simulink model "Combined_Experiment_Mar25_2020a_SpeedControl"  (R2020a)
settings: Solver=FixedStepAuto  StartTime=0.0  StopTime=tsim  FixedStep=baseRate  MaxStep=0.0001  RelTol=1e-6  AbsTol=1e-6  EnableMultiTasking=on
values from neighbouring files (symbols this model uses):
  b0 = importdata("biases_layer_0.csv")    [Run_Initializer.m]
  b1 = importdata("biases_layer_1.csv")    [Run_Initializer.m]
  b_out = importdata("biases_output.csv")    [Run_Initializer.m]
  baseRate = 0.05    [Run_Initializer.m]
  CHASER_ABSOLUTE_POSITION = true    [Run_Initializer.m]
  drop_states_ARM = [ pi/2, pi/2, 0]    [Run_Initializer.m]
  drop_states_BLACK = [ xLength/2, yLength/2, pi]    [Run_Initializer.m]
  drop_states_BLUE = [ xLength/2, yLength/2, pi]    [Run_Initializer.m]
  drop_states_RED = [ xLength/2+0.5, yLength/2, pi]    [Run_Initializer.m]
  F_Black_X_nominal = 0.2196    [Run_Initializer.m]
  F_Black_Y_nominal = 0.2825    [Run_Initializer.m]
  F_Blue_X_nominal = 0.2196    [Run_Initializer.m]
  F_Blue_Y_nominal = 0.2825    [Run_Initializer.m]
  F_red_X_nominal = 0.2196    [Run_Initializer.m]
  F_red_Y_nominal = 0.2825    [Run_Initializer.m]
  F_thrusters_BLACK = [F_Black_X_nominal; F_Black_X_nominal;                             F_Black_Y_nominal; F_Black_Y_nominal; F_Black_X_nominal;                              F_Black_X_nominal; F_Black_Y_nominal; F_Black_Y_nominal]    [Run_Initializer.m]
  F_thrusters_BLUE = [F_Blue_X_nominal; F_Blue_X_nominal;                             F_Blue_Y_nominal; F_Blue_Y_nominal; F_Blue_X_nominal;                              F_Blue_X_nominal; F_Blue_Y_nominal; F_Blue_Y_nominal]    [Run_Initializer.m]
  F_thrusters_RED = [F_red_X_nominal; F_red_X_nominal;                             F_red_Y_nominal; F_red_Y_nominal; F_red_X_nominal;                              F_red_X_nominal; F_red_Y_nominal; F_red_Y_nominal]    [Run_Initializer.m]
  Gamma1_el = 0.12    [Run_Initializer.m]
  Gamma1_sh = 0.005    [Run_Initializer.m]
  Gamma1_wr = 0.025    [Run_Initializer.m]
  Gamma2_el = 5    [Run_Initializer.m]
  Gamma2_sh = 15    [Run_Initializer.m]
  Gamma2_wr = 5    [Run_Initializer.m]
  Gamma3_el = 10    [Run_Initializer.m]
  Gamma3_sh = 40    [Run_Initializer.m]
  Gamma3_wr = 40    [Run_Initializer.m]
  Gamma4_el = 0.039    [Run_Initializer.m]
  Gamma4_sh = 0.015    [Run_Initializer.m]
  Gamma4_wr = 0.029    [Run_Initializer.m]
  Gamma5_el = 800    [Run_Initializer.m]
  Gamma5_sh = 800    [Run_Initializer.m]
  Gamma5_wr = 800    [Run_Initializer.m]
  Gamma6_el = 0.000001    (= 1e-06)    [Run_Initializer.m]
  Gamma6_sh = 0.005    [Run_Initializer.m]
  Gamma6_wr = 0.02    [Run_Initializer.m]
  HOLD_POINT_RADIUS = 0.95    [Run_Initializer.m]
  home_states_BLACK = [ xLength/2; yLength/2; 0]    [Run_Initializer.m]
  home_states_BLUE = [ xLength/2; yLength/2; 0]    [Run_Initializer.m]
  home_states_RED = [ xLength/2+0.9; yLength/2; pi]    [Run_Initializer.m]
  init_states_BLACK = [ xLength/2; yLength/2; pi]    [Run_Initializer.m]
  init_states_BLUE = [ xLength/2; yLength/2; pi]    [Run_Initializer.m]
  init_states_RED = [ xLength/2+0.9; yLength/2; pi]    [Run_Initializer.m]
  Kd_tb = 1.0    (= 1)    [Run_Initializer.m]
  Kd_tblue = 1    [Run_Initializer.m]
  Kd_tr = 1.0    (= 1)    [Run_Initializer.m]
  Kd_xb = 8    [Run_Initializer.m]
  Kd_xblue = 8    [Run_Initializer.m]
  Kd_xr = 8    [Run_Initializer.m]
  Kd_yb = 8    [Run_Initializer.m]
  Kd_yblue = 8    [Run_Initializer.m]
  Kd_yr = 8    [Run_Initializer.m]
  Kp_tb = 0.1    [Run_Initializer.m]
  Kp_tblue = 0.1    [Run_Initializer.m]
  Kp_tr = 0.1    [Run_Initializer.m]
  Kp_xb = 2    [Run_Initializer.m]
  Kp_xblue = 2    [Run_Initializer.m]
  Kp_xr = 2    [Run_Initializer.m]
  Kp_yb = 2    [Run_Initializer.m]
  Kp_yblue = 2    [Run_Initializer.m]
  Kp_yr = 2    [Run_Initializer.m]
  MAX_BODY_ANGULAR_VELOCITY = 15*180/pi    (= 859.436692696)    [Run_Initializer.m]
  MAX_VELOCITY = 0.1    [Run_Initializer.m]
  noise_variance_BLACK = 0    [Run_Initializer.m]
  noise_variance_BLUE = 0    [Run_Initializer.m]
  noise_variance_RED = 0    [Run_Initializer.m]
  Phase0_End = Phase0_Duration    (= 10)    [Run_Initializer.m]
  Phase1_End = Phase0_Duration + Phase1_Duration    (= 15)    [Run_Initializer.m]
  Phase2_End = Phase0_Duration + Phase1_Duration +                                   Phase2_Duration    (= 45)    [Run_Initializer.m]
  Phase3_End = Phase0_Duration + Phase1_Duration +                                   Phase2_Duration + Phase3_Duration    (= 560)    [Run_Initializer.m]
  Phase3_SubPhase1_End = Phase2_End + Phase3_SubPhase1_Duration    (= 105)    [Run_Initializer.m]
  Phase3_SubPhase2_End = Phase2_End + Phase3_SubPhase1_Duration +                                   Phase3_SubPhase2_Duration    (= 210)    [Run_Initializer.m]
  Phase3_SubPhase3_End = Phase2_End + Phase3_SubPhase1_Duration +                                   Phase3_SubPhase2_Duration +                                  Phase3_SubPhase3_Duration    (= 240)    [Run_Initializer.m]
  Phase3_SubPhase4_End = Phase2_End + Phase3_SubPhase1_Duration +                                   Phase3_SubPhase2_Duration +                                  Phase3_SubPhase3_Duration +                                  Phase3_SubPhase4_Duration    [Run_Initializer.m]
  Phase4_End = Phase0_Duration + Phase1_Duration +                                   Phase2_Duration + Phase3_Duration +                                   Phase4_Duration    (= 680)    [Run_Initializer.m]
  Phase5_End = Phase0_Duration + Phase1_Duration +                                   Phase2_Duration + Phase3_Duration +                                   Phase4_Duration + Phase5_Duration    (= 700)    [Run_Initializer.m]
  relevant_half_range = (upper_state_bound - lower_state_bound)/2    [Run_Initializer.m]
  relevant_state_mean = (lower_state_bound + upper_state_bound)/2    [Run_Initializer.m]
  thruster_dist2CG_BLACK = [72.80;-65.20;61.75;-79.75;65.20;-65.20;74.25;-54.75]    [Run_Initializer.m]
  thruster_dist2CG_BLUE = [83.10;-54.90;71.50;-70.00;54.90;-75.50;64.50;-64.50]    [Run_Initializer.m]
  thruster_dist2CG_RED = [69.38;-56.62;50.01;-81.49;61.12;-68.38;78.99;-52.01]    [Run_Initializer.m]
  w0 = importdata("weights_layer_0.csv")    [Run_Initializer.m]
  w1 = importdata("weights_layer_1.csv")    [Run_Initializer.m]
  w_out = importdata("weights_output.csv")    [Run_Initializer.m]
  xLength = 3.51155    [Run_Initializer.m]
  yLength = 2.41935    [Run_Initializer.m]
undefined symbols (not defined in the file or in its folder): DiscIntNeverNeededParam, model_param, platformSelection, serverRate, simMode
libraries: dspstat3 x18, raspberrypiBasiclib x9, dspsigops x9, simulink x8, embdlinuxlib x7, MainLibrary x4, mspfiltlib x3, dsparch4 x3, etargetslib x1, sensehatlib x1
(part 8 of 13)

== system Combined_Experiment_Mar25_2020a_SpeedControl/Phase #3: Experiment/Change RED Behavior/Sub-Phase #3 /RED+ARM ==
  note: ARM Control Law - RED
  note: This section is reserved for any control law for the robotic manipulator.
  Action Port : ActionPort  ActionPortLabel=if(u1 == 4 | u1 == 5 | u1 == 10 | u1 == 11)
  1-D Lookup Table : Lookup_n-D  NumberOfTableDimensions=1  BreakpointsForDimension1=|  Table=|  InternalRulePriority=Speed  RndMeth=Simplest  InputSameDT=on
      BreakpointsForDimension1=|
      | [0
      | 0.300000000000000
      | 0.600000000000000
      | 0.900000000000000
      | 1.20000000000000
      | 1.50000000000000
      | 1.80000000000000
      | 2.10000000000000
      | 2.40000000000000
      | 2.70000000000000
      | 3
      | 3.30000000000000
      | 3.60000000000000
      | 3.90000000000000
      | 4.20000000000000
      | 4.50000000000000
      | 4.80000000000000
      | 5.10000000000000
      | 5.40000000000000
      | 5.70000000000000
      | 6
      | 6.30000000000000
      | 6.60000000000000
      | 6.90000000000000
      | 7.20000000000000
      | 7.50000000000000
      | 7.80000000000000
      | 8.10000000000000
      | 8.40000000000000
      | 8.70000000000000
      | 9
      | 9.30000000000000
      | 9.60000000000000
      | 9.90000000000000
      | 10.2000000000000
      | 10.5000000000000
      | 10.8000000000000
      | 11.1000000000000
      | 11.4000000000000
      | 11.7000000000000
      | 12
      | 12.3000000000000
      | 12.6000000000000
      | 12.9000000000000
      | 13.2000000000000
      | 13.5000000000000
      | 13.8000000000000
      | 14.1000000000000
      | 14.4000000000000
      | 14.7000000000000
      | 15
      | 15.3000000000000
      | 15.6000000000000
      | 15.9000000000000
      | 16.2000000000000
      | 16.5000000000000
      | 16.8000000000000
      | 17.1000000000000
      | 17.4000000000000
      | 17.7000000000000
      | 18
      | 18.3000000000000
      | 18.6000000000000
      | 18.9000000000000
      | 19.2000000000000
      | 19.5000000000000
      | 19.8000000000000
      | 20.1000000000000
      | 20.4000000000000
      | 20.7000000000000
      | 21
      | 21.3000000000000
      | 21.6000000000000
      | 21.9000000000000
      | 22.2000000000000
      | 22.5000000000000
      | 22.8000000000000
      | 23.1000000000000
      | 23.4000000000000
      | 23.7000000000000
      | 24
      | 24.3000000000000
      | 24.6000000000000
      | 24.9000000000000
      | 25.2000000000000
      | 25.5000000000000
      | 25.8000000000000
      | 26.1000000000000
      | 26.4000000000000
      | 26.7000000000000
      | 27
      | 27.3000000000000
      | 27.6000000000000
      | 27.9000000000000
      | 28.2000000000000
      | 28.5000000000000
      | 28.8000000000000
      | 29.1000000000000
      | 29.4000000000000
      | 29.7000000000000
      | 30]
      Table=|
      | [1.57000000000000
      | 1.54816700100684
      | 1.49097838714515
      | 1.40738374526561
      | 1.30517963261499
      | 1.19037595061406
      | 1.06817443571262
      | 0.943755752477061
      | 0.821348547944454
      | 0.703746844506339
      | 0.593625926874354
      | 0.493661079760138
      | 0.406301951764504
      | 0.332150464577563
      | 0.270904238844892
      | 0.222254718367453
      | 0.185893346946205
      | 0.161510391400890
      | 0.148507079640713
      | 0.145619174532266
      | 0.151489118608687
      | 0.164759354403110
      | 0.184072324448674
      | 0.208070471278512
      | 0.235433340233479
      | 0.265163793185692
      | 0.296431328827974
      | 0.328406827894775
      | 0.360261171120541
      | 0.391165239239719
      | 0.420289912986756
      | 0.446835197706220
      | 0.470407808441224
      | 0.490913309071205
      | 0.508264171683338
      | 0.522372868364801
      | 0.533151871202771
      | 0.540513652284423
      | 0.544370683696935
      | 0.544708678506983
      | 0.541826697403650
      | 0.536107583537685
      | 0.527934180942696
      | 0.517689333652287
      | 0.505755885700064
      | 0.492516681119634
      | 0.478354564411779
      | 0.463677280032886
      | 0.448984347405091
      | 0.434796424940426
      | 0.421634171050923
      | 0.410018244148617
      | 0.400469302645538
      | 0.393508004953720
      | 0.389655009485195
      | 0.389318793355856
      | 0.392420798366228
      | 0.398750326166947
      | 0.408096675929411
      | 0.420249146825022
      | 0.434997038025178
      | 0.452129648701280
      | 0.471436276672662
      | 0.492577909508950
      | 0.514735652583953
      | 0.536978444975800
      | 0.558375225762617
      | 0.577994934022531
      | 0.594906508833669
      | 0.608178889274159
      | 0.616885200503004
      | 0.620279657398225
      | 0.617862923664403
      | 0.609153311284521
      | 0.593669132241562
      | 0.570928698518508
      | 0.540450322098342
      | 0.501754708369804
      | 0.454651142688837
      | 0.399508826722755
      | 0.336761216407457
      | 0.266841767678842
      | 0.190183936472810
      | 0.107221178725261
      | 0.0184637402812976
      | -0.0750305460272099
      | -0.171966007758580
      | -0.271046003976081
      | -0.370973893742981
      | -0.470452548764951
      | -0.568113490727538
      | -0.662442454298735
      | -0.751907371290790
      | -0.834976173515947
      | -0.910130221885170
      | -0.976013131751286
      | -1.03137619058426
      | -1.07497442671845
      | -1.10593044052833
      | -1.12417944460303
      | -1.20000000000000]
  1-D Lookup Table1 : Lookup_n-D  NumberOfTableDimensions=1  BreakpointsForDimension1=|  Table=|  InternalRulePriority=Speed  RndMeth=Simplest  InputSameDT=on
      BreakpointsForDimension1=|
      | [0
      | 0.300000000000000
      | 0.600000000000000
      | 0.900000000000000
      | 1.20000000000000
      | 1.50000000000000
      | 1.80000000000000
      | 2.10000000000000
      | 2.40000000000000
      | 2.70000000000000
      | 3
      | 3.30000000000000
      | 3.60000000000000
      | 3.90000000000000
      | 4.20000000000000
      | 4.50000000000000
      | 4.80000000000000
      | 5.10000000000000
      | 5.40000000000000
      | 5.70000000000000
      | 6
      | 6.30000000000000
      | 6.60000000000000
      | 6.90000000000000
      | 7.20000000000000
      | 7.50000000000000
      | 7.80000000000000
      | 8.10000000000000
      | 8.40000000000000
      | 8.70000000000000
      | 9
      | 9.30000000000000
      | 9.60000000000000
      | 9.90000000000000
      | 10.2000000000000
      | 10.5000000000000
      | 10.8000000000000
      | 11.1000000000000
      | 11.4000000000000
      | 11.7000000000000
      | 12
      | 12.3000000000000
      | 12.6000000000000
      | 12.9000000000000
      | 13.2000000000000
      | 13.5000000000000
      | 13.8000000000000
      | 14.1000000000000
      | 14.4000000000000
      | 14.7000000000000
      | 15
      | 15.3000000000000
      | 15.6000000000000
      | 15.9000000000000
      | 16.2000000000000
      | 16.5000000000000
      | 16.8000000000000
      | 17.1000000000000
      | 17.4000000000000
      | 17.7000000000000
      | 18
      | 18.3000000000000
      | 18.6000000000000
      | 18.9000000000000
      | 19.2000000000000
      | 19.5000000000000
      | 19.8000000000000
      | 20.1000000000000
      | 20.4000000000000
      | 20.7000000000000
      | 21
      | 21.3000000000000
      | 21.6000000000000
      | 21.9000000000000
      | 22.2000000000000
      | 22.5000000000000
      | 22.8000000000000
      | 23.1000000000000
      | 23.4000000000000
      | 23.7000000000000
      | 24
      | 24.3000000000000
      | 24.6000000000000
      | 24.9000000000000
      | 25.2000000000000
      | 25.5000000000000
      | 25.8000000000000
      | 26.1000000000000
      | 26.4000000000000
      | 26.7000000000000
      | 27
      | 27.3000000000000
      | 27.6000000000000
      | 27.9000000000000
      | 28.2000000000000
      | 28.5000000000000
      | 28.8000000000000
      | 29.1000000000000
      | 29.4000000000000
      | 29.7000000000000
      | 30]
      Table=|
      | [1.57000000000000
      | 1.57050205302399
      | 1.57012603662556
      | 1.56661162770156
      | 1.55794488562962
      | 1.54285929753597
      | 1.52042643744410
      | 1.48973080887809
      | 1.45048425411524
      | 1.40334397159352
      | 1.34904540279350
      | 1.28832398919572
      | 1.22195859634965
      | 1.15108368811919
      | 1.07700776270488
      | 1.00104050705195
      | 0.924491608105622
      | 0.848670299127955
      | 0.774774399465782
      | 0.703745216061739
      | 0.636488084287358
      | 0.573908339514172
      | 0.516911317113714
      | 0.466402352457517
      | 0.423202448662068
      | 0.387397731516399
      | 0.358695572215780
      | 0.336800200665272
      | 0.321415846769937
      | 0.312246740434836
      | 0.308997111565029
      | 0.311335869993361
      | 0.318438699519253
      | 0.329118863211428
      | 0.342181246399115
      | 0.356430734411547
      | 0.370672212577955
      | 0.383710566227569
      | 0.394350680689622
      | 0.401518359647600
      | 0.404656733001405
      | 0.403347252632020
      | 0.397171371877986
      | 0.385710544077849
      | 0.368546222570152
      | 0.345259860693440
      | 0.315432914518483
      | 0.278792464474893
      | 0.235602325706072
      | 0.186249942164213
      | 0.131122757801505
      | 0.0706082165701402
      | 0.00509376242231024
      | -0.0650331606897945
      | -0.139385108813982
      | -0.217505825480346
      | -0.298640304539486
      | -0.381952484472539
      | -0.466606302239867
      | -0.551765694801835
      | -0.636594599118806
      | -0.720256952151143
      | -0.801916690711806
      | -0.880723763116082
      | -0.955775800494991
      | -1.02615820551012
      | -1.09095638082305
      | -1.14925572909537
      | -1.20014165298867
      | -1.24269955516454
      | -1.27602769714638
      | -1.29978061439030
      | -1.31436988730625
      | -1.32026130853269
      | -1.31792067070809
      | -1.30781376647092
      | -1.29040638845964
      | -1.26616853457129
      | -1.23607724309064
      | -1.20209333571039
      | -1.16629053007224
      | -1.13074254381788
      | -1.09752309458901
      | -1.06870590002731
      | -1.04630359496360
      | -1.03189323418052
      | -1.02686268208325
      | -1.03259903268412
      | -1.05048937999544
      | -1.08191093831646
      | -1.12679451437392
      | -1.18211552054693
      | -1.24448846973170
      | -1.31052787482445
      | -1.37689087303085
      | -1.44074960138572
      | -1.49961795103105
      | -1.55095978791926
      | -1.58081445088490
      | -1.54996443310863
      | -1.48000000000000]
  1-D Lookup Table2 : Lookup_n-D  NumberOfTableDimensions=1  BreakpointsForDimension1=|  Table=|  InternalRulePriority=Speed  RndMeth=Simplest  InputSameDT=on
      BreakpointsForDimension1=|
      | [0
      | 0.300000000000000
      | 0.600000000000000
      | 0.900000000000000
      | 1.20000000000000
      | 1.50000000000000
      | 1.80000000000000
      | 2.10000000000000
      | 2.40000000000000
      | 2.70000000000000
      | 3
      | 3.30000000000000
      | 3.60000000000000
      | 3.90000000000000
      | 4.20000000000000
      | 4.50000000000000
      | 4.80000000000000
      | 5.10000000000000
      | 5.40000000000000
      | 5.70000000000000
      | 6
      | 6.30000000000000
      | 6.60000000000000
      | 6.90000000000000
      | 7.20000000000000
      | 7.50000000000000
      | 7.80000000000000
      | 8.10000000000000
      | 8.40000000000000
      | 8.70000000000000
      | 9
      | 9.30000000000000
      | 9.60000000000000
      | 9.90000000000000
      | 10.2000000000000
      | 10.5000000000000
      | 10.8000000000000
      | 11.1000000000000
      | 11.4000000000000
      | 11.7000000000000
      | 12
      | 12.3000000000000
      | 12.6000000000000
      | 12.9000000000000
      | 13.2000000000000
      | 13.5000000000000
      | 13.8000000000000
      | 14.1000000000000
      | 14.4000000000000
      | 14.7000000000000
      | 15
      | 15.3000000000000
      | 15.6000000000000
      | 15.9000000000000
      | 16.2000000000000
      | 16.5000000000000
      | 16.8000000000000
      | 17.1000000000000
      | 17.4000000000000
      | 17.7000000000000
      | 18
      | 18.3000000000000
      | 18.6000000000000
      | 18.9000000000000
      | 19.2000000000000
      | 19.5000000000000
      | 19.8000000000000
      | 20.1000000000000
      | 20.4000000000000
      | 20.7000000000000
      | 21
      | 21.3000000000000
      | 21.6000000000000
      | 21.9000000000000
      | 22.2000000000000
      | 22.5000000000000
      | 22.8000000000000
      | 23.1000000000000
      | 23.4000000000000
      | 23.7000000000000
      | 24
      | 24.3000000000000
      | 24.6000000000000
      | 24.9000000000000
      | 25.2000000000000
      | 25.5000000000000
      | 25.8000000000000
      | 26.1000000000000
      | 26.4000000000000
      | 26.7000000000000
      | 27
      | 27.3000000000000
      | 27.6000000000000
      | 27.9000000000000
      | 28.2000000000000
      | 28.5000000000000
      | 28.8000000000000
      | 29.1000000000000
      | 29.4000000000000
      | 29.7000000000000
      | 30]
      Table=|
      | [4.24105195407198e-14
      | 0.00792484586540242
      | 0.0289766808051712
      | 0.0591226460349239
      | 0.0945266677508536
      | 0.132723049258546
      | 0.171865961865416
      | 0.210118613330810
      | 0.245977670299252
      | 0.278442298917847
      | 0.306553255045181
      | 0.329351294539841
      | 0.345978769405532
      | 0.356409999236062
      | 0.361026479142565
      | 0.360212485455902
      | 0.354352294506931
      | 0.343830913350855
      | 0.329212797758318
      | 0.311475554957133
      | 0.291654729751521
      | 0.270785866945703
      | 0.249904511343898
      | 0.230046207750326
      | 0.212190891231227
      | 0.196833909602021
      | 0.184220855187696
      | 0.174595248907400
      | 0.168200611680283
      | 0.165280464425496
      | 0.166078328062186
      | 0.170819192753770
      | 0.179469276510222
      | 0.191804652485855
      | 0.207596998435017
      | 0.226617992112058
      | 0.248639311271326
      | 0.273432633667171
      | 0.300769637053943
      | 0.330372138422153
      | 0.361748634952746
      | 0.394350586665731
      | 0.427629452980086
      | 0.461036693314793
      | 0.494023767088832
      | 0.526042133721183
      | 0.556543253290674
      | 0.585013755003088
      | 0.611069892609436
      | 0.634357776934821
      | 0.654523518804344
      | 0.671213229043108
      | 0.684073018476216
      | 0.692748997928769
      | 0.696887278225870
      | 0.696239394653257
      | 0.691014582997561
      | 0.681546260210274
      | 0.668167845572800
      | 0.651212758366539
      | 0.631014417872893
      | 0.607906243373263
      | 0.582221655279522
      | 0.554401355144190
      | 0.525287277542556
      | 0.495815140112214
      | 0.466920660490759
      | 0.439539556315785
      | 0.414607545224887
      | 0.393060344855659
      | 0.375828988968287
      | 0.363641886942561
      | 0.356951692355833
      | 0.356191311825241
      | 0.361793651967925
      | 0.374191619401025
      | 0.393818120741680
      | 0.421102648855173
      | 0.456063090510969
      | 0.497918715134657
      | 0.545797145289127
      | 0.598826003537267
      | 0.656132912441967
      | 0.716845494566115
      | 0.780034633378752
      | 0.844366607241886
      | 0.908331957834384
      | 0.970420511226358
      | 1.02912209348792
      | 1.08292634428082
      | 1.13029561275212
      | 1.16963648628818
      | 1.19934874289962
      | 1.21783216059706
      | 1.22367347867057
      | 1.21771835926845
      | 1.20231148671538
      | 1.17980152164021
      | 1.14786929261614
      | 1.11
      | 1.11000000000000]
  Constant : Constant  Value=Phase3_SubPhase2_End
  Constant7 : Constant
  Data Store Read : DataStoreRead  DataStoreName=Univ_Time
  Data Store Write : DataStoreWrite  DataStoreName=RED_Shoulder_Command
  Data Store Write1 : DataStoreWrite  DataStoreName=RED_Elbow_Command
  Data Store Write2 : DataStoreWrite  DataStoreName=RED_Wrist_Command
  Data Store Write3 : DataStoreWrite  DataStoreName=RED_ARM_Control_Mode
  Subtract4 : Sum  Inputs=+-
  wires:
  Subtract4/1 -> 1-D Lookup Table2/1, 1-D Lookup Table1/1, 1-D Lookup Table/1
  Constant/1 -> Subtract4/2
  Data Store Read/1 -> Subtract4/1
  1-D Lookup Table/1 -> Data Store Write/1
  1-D Lookup Table2/1 -> Data Store Write2/1
  1-D Lookup Table1/1 -> Data Store Write1/1
  Constant7/1 -> Data Store Write3/1

== system Combined_Experiment_Mar25_2020a_SpeedControl/Phase #3: Experiment/Change RED Behavior/Sub-Phase #4/Custom Discrete PD (Attitude) ==
  ez : Inport
  Sum3 : Sum
  kd_tr : Gain  Gain=Kd_tr
  kp_tr : Gain  Gain=Kp_tr
  "x_dot -> x2" : Subsystem
  Tz : Outport  VectorParamsAs1DForOutWhenUnconnected=off
  wires:
  kd_tr/1 -> Sum3/1
  Sum3/1 -> Tz/1
  kp_tr/1 -> Sum3/2
  "x_dot -> x2"/1(dy(t)/dt) -> kd_tr/1
  ez/1 -> "x_dot -> x2"/1(y(t)), kp_tr/1

== system Combined_Experiment_Mar25_2020a_SpeedControl/Phase #3: Experiment/Change RED Behavior/Sub-Phase #4/Hough Control ==
  Ref : Inport
  Act : Inport  Port=2
  MATLAB Function2 : MATLAB Function  TreatAsAtomicUnit=on
  MATLAB Function3 : MATLAB Function  TreatAsAtomicUnit=on
  MATLAB Function4 : MATLAB Function  TreatAsAtomicUnit=on
  Subtract2 : Sum  Inputs=+-
  Err : Outport  VectorParamsAs1DForOutWhenUnconnected=off
  wires:
  MATLAB Function4/1(e_out) -> Err/1
  MATLAB Function2/1(Oy) -> MATLAB Function4/1(Oy)
  Subtract2/1 -> MATLAB Function4/2(e_in)
  MATLAB Function2/2(Ox) -> Subtract2/1
  Act/1 -> MATLAB Function3/1(z)
  Ref/1 -> MATLAB Function2/1(z)
  MATLAB Function3/1(Ox) -> Subtract2/2

== system Combined_Experiment_Mar25_2020a_SpeedControl/Phase #3: Experiment/Change RED Behavior/Sub-Phase #4/RED ==
  note: ARM Control Law - RED
  note: When the ARM is not in use, send zeros.
  Action Port : ActionPort  ActionPortLabel=else
  ARM_Desired_Rz_Elbow : DataStoreWrite  Commented=on  DataStoreName=ARM_Desired_Rz_Elbow
  ARM_Desired_Rz_Shoulder : DataStoreWrite  Commented=on  DataStoreName=ARM_Desired_Rz_Shoulder
  ARM_Desired_Rz_Wrist : DataStoreWrite  Commented=on  DataStoreName=ARM_Desired_Rz_Wrist
  Constant1 : Constant  Commented=on  Value=pi/2
  Constant7 : Constant  Commented=on  Value=0
  wires:
  Constant7/1 -> ARM_Desired_Rz_Wrist/1
  Constant1/1 -> ARM_Desired_Rz_Shoulder/1, ARM_Desired_Rz_Elbow/1

== system Combined_Experiment_Mar25_2020a_SpeedControl/Phase #3: Experiment/Change RED Behavior/Sub-Phase #4/RED+ARM ==
  note: ARM Control Law - RED
  note: This section is reserved for any control law for the robotic manipulator.
  Action Port : ActionPort  ActionPortLabel=if(u1 == 4 | u1 == 5 | u1 == 10 | u1 == 11)
  Constant : Constant  Value=Phase3_SubPhase3_End+10
  Data Store Read : DataStoreRead  DataStoreName=RED_Rz_Shoulder
  Data Store Read1 : DataStoreRead  DataStoreName=RED_Rz_Elbow
  Data Store Read2 : DataStoreRead  DataStoreName=RED_Rz_Wrist
  Data Store Write : DataStoreWrite  DataStoreName=RED_Shoulder_Command
  Data Store Write1 : DataStoreWrite  DataStoreName=RED_Elbow_Command
  Data Store Write2 : DataStoreWrite  DataStoreName=RED_Wrist_Command
  Data Store Write3 : DataStoreWrite  DataStoreName=RED_ARM_Control_Mode
  Demux : Demux  Outputs=3
  Demux1 : Demux  Outputs=3
  MATLAB Function : MATLAB Function  TreatAsAtomicUnit=on
  MATLAB Function1 : MATLAB Function  TreatAsAtomicUnit=on
  Mux : Mux  Inputs=3
  Mux2 : Mux  Inputs=2
  Mux3 : Mux  Inputs=3
  Mux4 : Mux  Inputs=3
  RED_Px : DataStoreRead  DataStoreName=RED_Px
  RED_Px1 : DataStoreRead  DataStoreName=BLUE_Px
  "RED_Py " : DataStoreRead  DataStoreName=RED_Py
  RED_Py 1 : DataStoreRead  DataStoreName=BLUE_Py
  RED_Rz : DataStoreRead  DataStoreName=RED_Rz
  RED_Rz1 : DataStoreRead  DataStoreName=BLUE_Rz
  Subtract4 : Sum  Inputs=+-
  Terminator : Terminator
  Time : DataStoreRead  DataStoreName=Univ_Time
  Transpose Jacobian Controller : Subsystem
  wires:
  Demux1/2 -> Data Store Write1/1
  Demux1/1 -> Data Store Write/1
  MATLAB Function1/1(Control_Mode) -> Data Store Write3/1
  Demux1/3 -> Data Store Write2/1
  Mux2/1 -> Transpose Jacobian Controller/1(Ref)
  Data Store Read2/1 -> Mux3/3
  Data Store Read1/1 -> Mux3/2
  Data Store Read/1 -> Mux3/1
  Mux3/1 -> Transpose Jacobian Controller/2(q)
  MATLAB Function/1(p_red_target) -> Demux/1
  Demux/3 -> Terminator/1
  Demux/1 -> Mux2/1
  Demux/2 -> Mux2/2
  Transpose Jacobian Controller/1(Control) -> Demux1/1
  RED_Px/1 -> Mux/1
  "RED_Py "/1 -> Mux/2
  RED_Rz/1 -> Mux/3
  Mux/1 -> MATLAB Function/1(RED)
  RED_Px1/1 -> Mux4/1
  RED_Py 1/1 -> Mux4/2
  RED_Rz1/1 -> Mux4/3
  Mux4/1 -> MATLAB Function/2(BLACK)
  Time/1 -> Subtract4/1
  Constant/1 -> Subtract4/2
  Subtract4/1 -> MATLAB Function1/1(Sim_Time)

== system Combined_Experiment_Mar25_2020a_SpeedControl/Phase #4: Return Home/Change BLACK Behavior/Custom Discrete PD (Attitude)/x_dot -> x1 ==
  note: dy/dt ~= (y2-y1)/deltaT
  y(t) : Inport
  Delay1 : Delay  DelayLength=1  InitialConditionSource=Input port
      settings: InputPortMap=u0,p4
  Hold this value : Subsystem  TreatAsAtomicUnit=on
  Sum6 : Sum  Inputs=-+|
  divide by delta T : Gain  Gain=1/baseRate
  "if we went through a \"step\"" : If  IfExpression=u1 ~= 0  ShowElse=off
  dy(t)/dt : Outport  VectorParamsAs1DForOutWhenUnconnected=off
  wires:
  divide by delta T/1 -> dy(t)/dt/1
  Delay1/1 -> Sum6/1
  "if we went through a \"step\""/1 -> Hold this value/Action
  Hold this value/1(Out1) -> divide by delta T/1
  Sum6/1 -> "if we went through a \"step\""/1, Hold this value/1(In1)
  y(t)/1 -> Sum6/2, Delay1/2, Delay1/1

== system Combined_Experiment_Mar25_2020a_SpeedControl/Phase #4: Return Home/Change BLACK Behavior/Custom Discrete PD (X-Position)/x_dot -> x1 ==
  note: dy/dt ~= (y2-y1)/deltaT
  y(t) : Inport
  Delay1 : Delay  DelayLength=1  InitialConditionSource=Input port
      settings: InputPortMap=u0,p4
  Hold this value : Subsystem  TreatAsAtomicUnit=on
  Sum6 : Sum  Inputs=-+|
  divide by delta T : Gain  Gain=1/baseRate
  "if we went through a \"step\"" : If  IfExpression=u1 ~= 0  ShowElse=off
  dy(t)/dt : Outport  VectorParamsAs1DForOutWhenUnconnected=off
  wires:
  divide by delta T/1 -> dy(t)/dt/1
  Delay1/1 -> Sum6/1
  "if we went through a \"step\""/1 -> Hold this value/Action
  Hold this value/1(Out1) -> divide by delta T/1
  Sum6/1 -> "if we went through a \"step\""/1, Hold this value/1(In1)
  y(t)/1 -> Sum6/2, Delay1/2, Delay1/1

== system Combined_Experiment_Mar25_2020a_SpeedControl/Phase #4: Return Home/Change BLACK Behavior/Custom Discrete PD (Y-Position)/x_dot -> x1 ==
  note: dy/dt ~= (y2-y1)/deltaT
  y(t) : Inport
  Delay1 : Delay  DelayLength=1  InitialConditionSource=Input port
      settings: InputPortMap=u0,p4
  Hold this value : Subsystem  TreatAsAtomicUnit=on
  Sum6 : Sum  Inputs=-+|
  divide by delta T : Gain  Gain=1/baseRate
  "if we went through a \"step\"" : If  IfExpression=u1 ~= 0  ShowElse=off
  dy(t)/dt : Outport  VectorParamsAs1DForOutWhenUnconnected=off
  wires:
  divide by delta T/1 -> dy(t)/dt/1
  Delay1/1 -> Sum6/1
  "if we went through a \"step\""/1 -> Hold this value/Action
  Hold this value/1(Out1) -> divide by delta T/1
  Sum6/1 -> "if we went through a \"step\""/1, Hold this value/1(In1)
  y(t)/1 -> Sum6/2, Delay1/2, Delay1/1

== system Combined_Experiment_Mar25_2020a_SpeedControl/Phase #4: Return Home/Change BLUE Behavior/Custom Discrete PD (Attitude)/x_dot -> x1 ==
  note: dy/dt ~= (y2-y1)/deltaT
  y(t) : Inport
  Delay1 : Delay  DelayLength=1  InitialConditionSource=Input port
      settings: InputPortMap=u0,p4
  Hold this value : Subsystem  TreatAsAtomicUnit=on
  Sum6 : Sum  Inputs=-+|
  divide by delta T : Gain  Gain=1/baseRate
  "if we went through a \"step\"" : If  IfExpression=u1 ~= 0  ShowElse=off
  dy(t)/dt : Outport  VectorParamsAs1DForOutWhenUnconnected=off
  wires:
  divide by delta T/1 -> dy(t)/dt/1
  Delay1/1 -> Sum6/1
  "if we went through a \"step\""/1 -> Hold this value/Action
  Hold this value/1(Out1) -> divide by delta T/1
  Sum6/1 -> "if we went through a \"step\""/1, Hold this value/1(In1)
  y(t)/1 -> Sum6/2, Delay1/2, Delay1/1

== system Combined_Experiment_Mar25_2020a_SpeedControl/Phase #4: Return Home/Change BLUE Behavior/Custom Discrete PD (X-Position)/x_dot -> x1 ==
  note: dy/dt ~= (y2-y1)/deltaT
  y(t) : Inport
  Delay1 : Delay  DelayLength=1  InitialConditionSource=Input port
      settings: InputPortMap=u0,p4
  Hold this value : Subsystem  TreatAsAtomicUnit=on
  Sum6 : Sum  Inputs=-+|
  divide by delta T : Gain  Gain=1/baseRate
  "if we went through a \"step\"" : If  IfExpression=u1 ~= 0  ShowElse=off
  dy(t)/dt : Outport  VectorParamsAs1DForOutWhenUnconnected=off
  wires:
  divide by delta T/1 -> dy(t)/dt/1
  Delay1/1 -> Sum6/1
  "if we went through a \"step\""/1 -> Hold this value/Action
  Hold this value/1(Out1) -> divide by delta T/1
  Sum6/1 -> "if we went through a \"step\""/1, Hold this value/1(In1)
  y(t)/1 -> Sum6/2, Delay1/2, Delay1/1

== system Combined_Experiment_Mar25_2020a_SpeedControl/Phase #4: Return Home/Change BLUE Behavior/Custom Discrete PD (Y-Position)/x_dot -> x1 ==
  note: dy/dt ~= (y2-y1)/deltaT
  y(t) : Inport
  Delay1 : Delay  DelayLength=1  InitialConditionSource=Input port
      settings: InputPortMap=u0,p4
  Hold this value : Subsystem  TreatAsAtomicUnit=on
  Sum6 : Sum  Inputs=-+|
  divide by delta T : Gain  Gain=1/baseRate
  "if we went through a \"step\"" : If  IfExpression=u1 ~= 0  ShowElse=off
  dy(t)/dt : Outport  VectorParamsAs1DForOutWhenUnconnected=off
  wires:
  divide by delta T/1 -> dy(t)/dt/1
  Delay1/1 -> Sum6/1
  "if we went through a \"step\""/1 -> Hold this value/Action
  Hold this value/1(Out1) -> divide by delta T/1
  Sum6/1 -> "if we went through a \"step\""/1, Hold this value/1(In1)
  y(t)/1 -> Sum6/2, Delay1/2, Delay1/1

== system Combined_Experiment_Mar25_2020a_SpeedControl/Phase #4: Return Home/Change RED Behavior/Custom Discrete PD (Attitude)/x_dot -> x2 ==
  note: dy/dt ~= (y2-y1)/deltaT
  y(t) : Inport
  Delay1 : Delay  DelayLength=1  InitialConditionSource=Input port
      settings: InputPortMap=u0,p4
  Hold this value : Subsystem  TreatAsAtomicUnit=on
  Sum6 : Sum  Inputs=-+|
  divide by delta T : Gain  Gain=1/baseRate
  "if we went through a \"step\"" : If  IfExpression=u1 ~= 0  ShowElse=off
  dy(t)/dt : Outport  VectorParamsAs1DForOutWhenUnconnected=off
  wires:
  divide by delta T/1 -> dy(t)/dt/1
  Delay1/1 -> Sum6/1
  "if we went through a \"step\""/1 -> Hold this value/Action
  Hold this value/1(Out1) -> divide by delta T/1
  Sum6/1 -> "if we went through a \"step\""/1, Hold this value/1(In1)
  y(t)/1 -> Sum6/2, Delay1/2, Delay1/1

== system Combined_Experiment_Mar25_2020a_SpeedControl/Phase #4: Return Home/Change RED Behavior/Custom Discrete PD (X-Position)/x_dot -> x2 ==
  note: dy/dt ~= (y2-y1)/deltaT
  y(t) : Inport
  Delay1 : Delay  DelayLength=1  InitialConditionSource=Input port
      settings: InputPortMap=u0,p4
  Hold this value : Subsystem  TreatAsAtomicUnit=on
  Sum6 : Sum  Inputs=-+|
  divide by delta T : Gain  Gain=1/baseRate
  "if we went through a \"step\"" : If  IfExpression=u1 ~= 0  ShowElse=off
  dy(t)/dt : Outport  VectorParamsAs1DForOutWhenUnconnected=off
  wires:
  divide by delta T/1 -> dy(t)/dt/1
  Delay1/1 -> Sum6/1
  "if we went through a \"step\""/1 -> Hold this value/Action
  Hold this value/1(Out1) -> divide by delta T/1
  Sum6/1 -> "if we went through a \"step\""/1, Hold this value/1(In1)
  y(t)/1 -> Sum6/2, Delay1/2, Delay1/1

== system Combined_Experiment_Mar25_2020a_SpeedControl/Phase #4: Return Home/Change RED Behavior/Custom Discrete PD (Y-Position)/x_dot -> x2 ==
  note: dy/dt ~= (y2-y1)/deltaT
  y(t) : Inport
  Delay1 : Delay  DelayLength=1  InitialConditionSource=Input port
      settings: InputPortMap=u0,p4
  Hold this value : Subsystem  TreatAsAtomicUnit=on
  Sum6 : Sum  Inputs=-+|
  divide by delta T : Gain  Gain=1/baseRate
  "if we went through a \"step\"" : If  IfExpression=u1 ~= 0  ShowElse=off
  dy(t)/dt : Outport  VectorParamsAs1DForOutWhenUnconnected=off
  wires:
  divide by delta T/1 -> dy(t)/dt/1
  Delay1/1 -> Sum6/1
  "if we went through a \"step\""/1 -> Hold this value/Action
  Hold this value/1(Out1) -> divide by delta T/1
  Sum6/1 -> "if we went through a \"step\""/1, Hold this value/1(In1)
  y(t)/1 -> Sum6/2, Delay1/2, Delay1/1

== system Combined_Experiment_Mar25_2020a_SpeedControl/Phase #5: Hold Home/Change BLACK Behavior/Custom Discrete PD (Attitude)/x_dot -> x1 ==
  note: dy/dt ~= (y2-y1)/deltaT
  y(t) : Inport
  Delay1 : Delay  DelayLength=1  InitialConditionSource=Input port
      settings: InputPortMap=u0,p4
  Hold this value : Subsystem  TreatAsAtomicUnit=on
  Sum6 : Sum  Inputs=-+|
  divide by delta T : Gain  Gain=1/baseRate
  "if we went through a \"step\"" : If  IfExpression=u1 ~= 0  ShowElse=off
  dy(t)/dt : Outport  VectorParamsAs1DForOutWhenUnconnected=off
  wires:
  divide by delta T/1 -> dy(t)/dt/1
  Delay1/1 -> Sum6/1
  "if we went through a \"step\""/1 -> Hold this value/Action
  Hold this value/1(Out1) -> divide by delta T/1
  Sum6/1 -> "if we went through a \"step\""/1, Hold this value/1(In1)
  y(t)/1 -> Sum6/2, Delay1/2, Delay1/1

== system Combined_Experiment_Mar25_2020a_SpeedControl/Phase #5: Hold Home/Change BLACK Behavior/Custom Discrete PD (X-Position)/x_dot -> x1 ==
  note: dy/dt ~= (y2-y1)/deltaT
  y(t) : Inport
  Delay1 : Delay  DelayLength=1  InitialConditionSource=Input port
      settings: InputPortMap=u0,p4
  Hold this value : Subsystem  TreatAsAtomicUnit=on
  Sum6 : Sum  Inputs=-+|
  divide by delta T : Gain  Gain=1/baseRate
  "if we went through a \"step\"" : If  IfExpression=u1 ~= 0  ShowElse=off
  dy(t)/dt : Outport  VectorParamsAs1DForOutWhenUnconnected=off
  wires:
  divide by delta T/1 -> dy(t)/dt/1
  Delay1/1 -> Sum6/1
  "if we went through a \"step\""/1 -> Hold this value/Action
  Hold this value/1(Out1) -> divide by delta T/1
  Sum6/1 -> "if we went through a \"step\""/1, Hold this value/1(In1)
  y(t)/1 -> Sum6/2, Delay1/2, Delay1/1

== system Combined_Experiment_Mar25_2020a_SpeedControl/Phase #5: Hold Home/Change BLACK Behavior/Custom Discrete PD (Y-Position)/x_dot -> x1 ==
  note: dy/dt ~= (y2-y1)/deltaT
  y(t) : Inport
  Delay1 : Delay  DelayLength=1  InitialConditionSource=Input port
      settings: InputPortMap=u0,p4
  Hold this value : Subsystem  TreatAsAtomicUnit=on
  Sum6 : Sum  Inputs=-+|
  divide by delta T : Gain  Gain=1/baseRate
  "if we went through a \"step\"" : If  IfExpression=u1 ~= 0  ShowElse=off
  dy(t)/dt : Outport  VectorParamsAs1DForOutWhenUnconnected=off
  wires:
  divide by delta T/1 -> dy(t)/dt/1
  Delay1/1 -> Sum6/1
  "if we went through a \"step\""/1 -> Hold this value/Action
  Hold this value/1(Out1) -> divide by delta T/1
  Sum6/1 -> "if we went through a \"step\""/1, Hold this value/1(In1)
  y(t)/1 -> Sum6/2, Delay1/2, Delay1/1

== system Combined_Experiment_Mar25_2020a_SpeedControl/Phase #5: Hold Home/Change BLUE Behavior/Custom Discrete PD (Attitude)/x_dot -> x1 ==
  note: dy/dt ~= (y2-y1)/deltaT
  y(t) : Inport
  Delay1 : Delay  DelayLength=1  InitialConditionSource=Input port
      settings: InputPortMap=u0,p4
  Hold this value : Subsystem  TreatAsAtomicUnit=on
  Sum6 : Sum  Inputs=-+|
  divide by delta T : Gain  Gain=1/baseRate
  "if we went through a \"step\"" : If  IfExpression=u1 ~= 0  ShowElse=off
  dy(t)/dt : Outport  VectorParamsAs1DForOutWhenUnconnected=off
  wires:
  divide by delta T/1 -> dy(t)/dt/1
  Delay1/1 -> Sum6/1
  "if we went through a \"step\""/1 -> Hold this value/Action
  Hold this value/1(Out1) -> divide by delta T/1
  Sum6/1 -> "if we went through a \"step\""/1, Hold this value/1(In1)
  y(t)/1 -> Sum6/2, Delay1/2, Delay1/1

== system Combined_Experiment_Mar25_2020a_SpeedControl/Phase #5: Hold Home/Change BLUE Behavior/Custom Discrete PD (X-Position)/x_dot -> x1 ==
  note: dy/dt ~= (y2-y1)/deltaT
  y(t) : Inport
  Delay1 : Delay  DelayLength=1  InitialConditionSource=Input port
      settings: InputPortMap=u0,p4
  Hold this value : Subsystem  TreatAsAtomicUnit=on
  Sum6 : Sum  Inputs=-+|
  divide by delta T : Gain  Gain=1/baseRate
  "if we went through a \"step\"" : If  IfExpression=u1 ~= 0  ShowElse=off
  dy(t)/dt : Outport  VectorParamsAs1DForOutWhenUnconnected=off
  wires:
  divide by delta T/1 -> dy(t)/dt/1
  Delay1/1 -> Sum6/1
  "if we went through a \"step\""/1 -> Hold this value/Action
  Hold this value/1(Out1) -> divide by delta T/1
  Sum6/1 -> "if we went through a \"step\""/1, Hold this value/1(In1)
  y(t)/1 -> Sum6/2, Delay1/2, Delay1/1

== system Combined_Experiment_Mar25_2020a_SpeedControl/Phase #5: Hold Home/Change BLUE Behavior/Custom Discrete PD (Y-Position)/x_dot -> x1 ==
  note: dy/dt ~= (y2-y1)/deltaT
  y(t) : Inport
  Delay1 : Delay  DelayLength=1  InitialConditionSource=Input port
      settings: InputPortMap=u0,p4
  Hold this value : Subsystem  TreatAsAtomicUnit=on
  Sum6 : Sum  Inputs=-+|
  divide by delta T : Gain  Gain=1/baseRate
  "if we went through a \"step\"" : If  IfExpression=u1 ~= 0  ShowElse=off
  dy(t)/dt : Outport  VectorParamsAs1DForOutWhenUnconnected=off
  wires:
  divide by delta T/1 -> dy(t)/dt/1
  Delay1/1 -> Sum6/1
  "if we went through a \"step\""/1 -> Hold this value/Action
  Hold this value/1(Out1) -> divide by delta T/1
  Sum6/1 -> "if we went through a \"step\""/1, Hold this value/1(In1)
  y(t)/1 -> Sum6/2, Delay1/2, Delay1/1

== system Combined_Experiment_Mar25_2020a_SpeedControl/Phase #5: Hold Home/Change RED Behavior/Custom Discrete PD (Attitude)/x_dot -> x2 ==
  note: dy/dt ~= (y2-y1)/deltaT
  y(t) : Inport
  Delay1 : Delay  DelayLength=1  InitialConditionSource=Input port
      settings: InputPortMap=u0,p4
  Hold this value : Subsystem  TreatAsAtomicUnit=on
  Sum6 : Sum  Inputs=-+|
  divide by delta T : Gain  Gain=1/baseRate
  "if we went through a \"step\"" : If  IfExpression=u1 ~= 0  ShowElse=off
  dy(t)/dt : Outport  VectorParamsAs1DForOutWhenUnconnected=off
  wires:
  divide by delta T/1 -> dy(t)/dt/1
  Delay1/1 -> Sum6/1
  "if we went through a \"step\""/1 -> Hold this value/Action
  Hold this value/1(Out1) -> divide by delta T/1
  Sum6/1 -> "if we went through a \"step\""/1, Hold this value/1(In1)
  y(t)/1 -> Sum6/2, Delay1/2, Delay1/1

== system Combined_Experiment_Mar25_2020a_SpeedControl/Phase #5: Hold Home/Change RED Behavior/Custom Discrete PD (X-Position)/x_dot -> x2 ==
  note: dy/dt ~= (y2-y1)/deltaT
  y(t) : Inport
  Delay1 : Delay  DelayLength=1  InitialConditionSource=Input port
      settings: InputPortMap=u0,p4
  Hold this value : Subsystem  TreatAsAtomicUnit=on
  Sum6 : Sum  Inputs=-+|
  divide by delta T : Gain  Gain=1/baseRate
  "if we went through a \"step\"" : If  IfExpression=u1 ~= 0  ShowElse=off
  dy(t)/dt : Outport  VectorParamsAs1DForOutWhenUnconnected=off
  wires:
  divide by delta T/1 -> dy(t)/dt/1
  Delay1/1 -> Sum6/1
  "if we went through a \"step\""/1 -> Hold this value/Action
  Hold this value/1(Out1) -> divide by delta T/1
  Sum6/1 -> "if we went through a \"step\""/1, Hold this value/1(In1)
  y(t)/1 -> Sum6/2, Delay1/2, Delay1/1

== system Combined_Experiment_Mar25_2020a_SpeedControl/Phase #5: Hold Home/Change RED Behavior/Custom Discrete PD (Y-Position)/x_dot -> x2 ==
  note: dy/dt ~= (y2-y1)/deltaT
  y(t) : Inport
  Delay1 : Delay  DelayLength=1  InitialConditionSource=Input port
      settings: InputPortMap=u0,p4
  Hold this value : Subsystem  TreatAsAtomicUnit=on
  Sum6 : Sum  Inputs=-+|
  divide by delta T : Gain  Gain=1/baseRate
  "if we went through a \"step\"" : If  IfExpression=u1 ~= 0  ShowElse=off
  dy(t)/dt : Outport  VectorParamsAs1DForOutWhenUnconnected=off
  wires:
  divide by delta T/1 -> dy(t)/dt/1
  Delay1/1 -> Sum6/1
  "if we went through a \"step\""/1 -> Hold this value/Action
  Hold this value/1(Out1) -> divide by delta T/1
  Sum6/1 -> "if we went through a \"step\""/1, Hold this value/1(In1)
  y(t)/1 -> Sum6/2, Delay1/2, Delay1/1

== system Combined_Experiment_Mar25_2020a_SpeedControl/Simulate Plant Dynamics/BLACK Dynamics/x_dot -> x1/Hold this value ==
  In1 : Inport
  Action Port : ActionPort  ActionPortLabel=if(u1 ~= 0)
  Out1 : Outport  VectorParamsAs1DForOutWhenUnconnected=off
  wires:
  In1/1 -> Out1/1

== system Combined_Experiment_Mar25_2020a_SpeedControl/Simulate Plant Dynamics/BLACK Dynamics/x_dot -> x2/Hold this value ==
  In1 : Inport
  Action Port : ActionPort  ActionPortLabel=if(u1 ~= 0)
  Out1 : Outport  VectorParamsAs1DForOutWhenUnconnected=off
  wires:
  In1/1 -> Out1/1

== system Combined_Experiment_Mar25_2020a_SpeedControl/Simulate Plant Dynamics/BLACK Dynamics/x_dot -> x3/Hold this value ==
  In1 : Inport
  Action Port : ActionPort  ActionPortLabel=if(u1 ~= 0)
  Out1 : Outport  VectorParamsAs1DForOutWhenUnconnected=off
  wires:
  In1/1 -> Out1/1

== system Combined_Experiment_Mar25_2020a_SpeedControl/Simulate Plant Dynamics/BLACK Dynamics/x_dot -> x4/Hold this value ==
  In1 : Inport
  Action Port : ActionPort  ActionPortLabel=if(u1 ~= 0)
  Out1 : Outport  VectorParamsAs1DForOutWhenUnconnected=off
  wires:
  In1/1 -> Out1/1

== system Combined_Experiment_Mar25_2020a_SpeedControl/Simulate Plant Dynamics/BLACK Dynamics/x_dot -> x7/Hold this value ==
  In1 : Inport
  Action Port : ActionPort  ActionPortLabel=if(u1 ~= 0)
  Out1 : Outport  VectorParamsAs1DForOutWhenUnconnected=off
  wires:
  In1/1 -> Out1/1

== system Combined_Experiment_Mar25_2020a_SpeedControl/Simulate Plant Dynamics/BLUE Dynamics/x_dot -> x1/Hold this value ==
  In1 : Inport
  Action Port : ActionPort  ActionPortLabel=if(u1 ~= 0)
  Out1 : Outport  VectorParamsAs1DForOutWhenUnconnected=off
  wires:
  In1/1 -> Out1/1

== system Combined_Experiment_Mar25_2020a_SpeedControl/Simulate Plant Dynamics/BLUE Dynamics/x_dot -> x2/Hold this value ==
  In1 : Inport
  Action Port : ActionPort  ActionPortLabel=if(u1 ~= 0)
  Out1 : Outport  VectorParamsAs1DForOutWhenUnconnected=off
  wires:
  In1/1 -> Out1/1

== system Combined_Experiment_Mar25_2020a_SpeedControl/Simulate Plant Dynamics/BLUE Dynamics/x_dot -> x3/Hold this value ==
  In1 : Inport
  Action Port : ActionPort  ActionPortLabel=if(u1 ~= 0)
  Out1 : Outport  VectorParamsAs1DForOutWhenUnconnected=off
  wires:
  In1/1 -> Out1/1

== system Combined_Experiment_Mar25_2020a_SpeedControl/Simulate Plant Dynamics/BLUE Dynamics/x_dot -> x4/Hold this value ==
  In1 : Inport
  Action Port : ActionPort  ActionPortLabel=if(u1 ~= 0)
  Out1 : Outport  VectorParamsAs1DForOutWhenUnconnected=off
  wires:
  In1/1 -> Out1/1

== system Combined_Experiment_Mar25_2020a_SpeedControl/Simulate Plant Dynamics/BLUE Dynamics/x_dot -> x7/Hold this value ==
  In1 : Inport
  Action Port : ActionPort  ActionPortLabel=if(u1 ~= 0)
  Out1 : Outport  VectorParamsAs1DForOutWhenUnconnected=off
  wires:
  In1/1 -> Out1/1

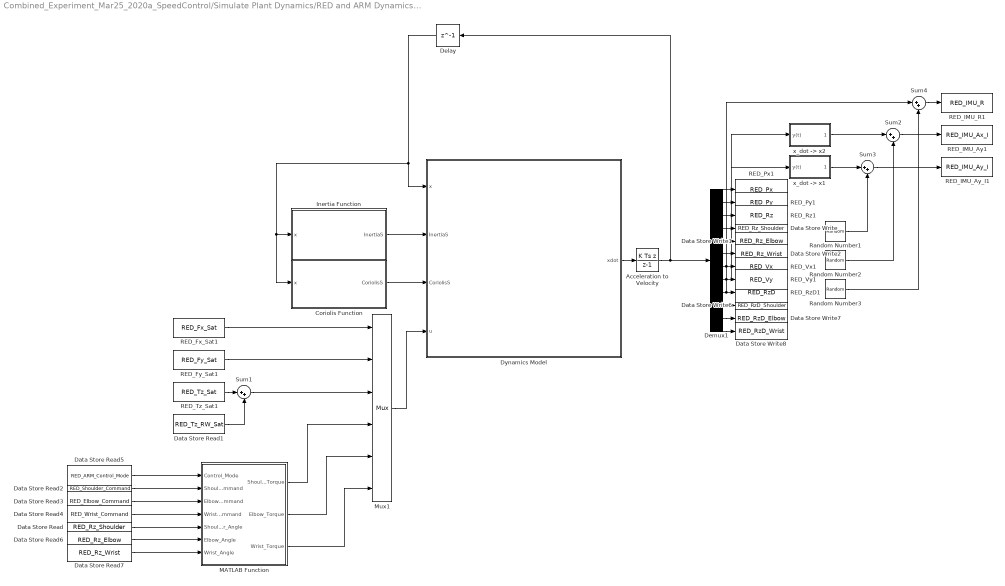
== system Combined_Experiment_Mar25_2020a_SpeedControl/Simulate Plant Dynamics/RED and ARM Dynamics/RED + ARM/RED + ARM Dynamics ==
  Acceleration to Velocity : DiscreteIntegrator  IntegratorMethod=Integration: Backward Euler  InitialCondition=[drop_states_RED,drop_states_ARM,0,0,0,0,0,0]  SampleTime=-1  ICPrevOutput=DiscIntNeverNeededParam  ICPrevScaledInput=DiscIntNeverNeededParam
  Coriolis Function : MATLAB Function  TreatAsAtomicUnit=on
  Data Store Read : DataStoreRead  DataStoreName=RED_Rz_Shoulder
  Data Store Read1 : DataStoreRead  DataStoreName=RED_Tz_RW_Sat
  Data Store Read2 : DataStoreRead  DataStoreName=RED_Shoulder_Command
  Data Store Read3 : DataStoreRead  DataStoreName=RED_Elbow_Command
  Data Store Read4 : DataStoreRead  DataStoreName=RED_Wrist_Command
  Data Store Read5 : DataStoreRead  DataStoreName=RED_ARM_Control_Mode
  Data Store Read6 : DataStoreRead  DataStoreName=RED_Rz_Elbow
  Data Store Read7 : DataStoreRead  DataStoreName=RED_Rz_Wrist
  Data Store Write : DataStoreWrite  DataStoreName=RED_Rz_Shoulder
  Data Store Write1 : DataStoreWrite  DataStoreName=RED_Rz_Elbow
  Data Store Write2 : DataStoreWrite  DataStoreName=RED_Rz_Wrist
  Data Store Write6 : DataStoreWrite  DataStoreName=RED_RzD_Shoulder
  Data Store Write7 : DataStoreWrite  DataStoreName=RED_RzD_Elbow
  Data Store Write8 : DataStoreWrite  DataStoreName=RED_RzD_Wrist
  Delay : Delay  DelayLength=1
  Demux1 : Demux  Outputs=12
  Dynamics Model : MATLAB Function  TreatAsAtomicUnit=on
  "Inertia Function " : MATLAB Function  TreatAsAtomicUnit=on
  MATLAB Function : MATLAB Function  TreatAsAtomicUnit=on
  Mux1 : Mux  Inputs=6
  RED_Fx_Sat1 : DataStoreRead  DataStoreName=RED_Fx_Sat
  RED_Fy_Sat1 : DataStoreRead  DataStoreName=RED_Fy_Sat
  RED_IMU_Ay1 : DataStoreWrite  DataStoreName=RED_IMU_Ax_I
  RED_IMU_Ay_I1 : DataStoreWrite  DataStoreName=RED_IMU_Ay_I
  RED_IMU_R1 : DataStoreWrite  DataStoreName=RED_IMU_R
  RED_Px1 : DataStoreWrite  DataStoreName=RED_Px
  RED_Py1 : DataStoreWrite  DataStoreName=RED_Py
  RED_Rz1 : DataStoreWrite  DataStoreName=RED_Rz
  RED_RzD1 : DataStoreWrite  DataStoreName=RED_RzD
  RED_Tz_Sat1 : DataStoreRead  DataStoreName=RED_Tz_Sat
  RED_Vx1 : DataStoreWrite  DataStoreName=RED_Vx
  RED_Vy1 : DataStoreWrite  DataStoreName=RED_Vy
  Random Number1 : RandomNumber  Variance=0
  Random Number2 : RandomNumber  Variance=0
  Random Number3 : RandomNumber  Variance=0
  Sum{1..4} (4 alike) : Sum  Inputs=|++
  "x_dot -> x1" : Subsystem
  "x_dot -> x2" : Subsystem
  wires:
  Mux1/1 -> Dynamics Model/4(u)
  Demux1/1 -> RED_Px1/1
  Demux1/2 -> RED_Py1/1
  Demux1/3 -> RED_Rz1/1
  Demux1/4 -> Data Store Write/1
  Demux1/5 -> Data Store Write1/1
  Demux1/6 -> Data Store Write2/1
  Demux1/7 -> "x_dot -> x2"/1(y(t)), RED_Vx1/1
  Demux1/9 -> Sum4/1, RED_RzD1/1
  Demux1/11 -> Data Store Write7/1
  RED_Tz_Sat1/1 -> Sum1/1
  Data Store Read1/1 -> Sum1/2
  Sum1/1 -> Mux1/3
  RED_Fx_Sat1/1 -> Mux1/1
  RED_Fy_Sat1/1 -> Mux1/2
  Sum2/1 -> RED_IMU_Ay1/1
  Random Number1/1 -> Sum3/2
  Random Number2/1 -> Sum2/2
  Sum3/1 -> RED_IMU_Ay_I1/1
  "x_dot -> x1"/1(dy(t)/dt) -> Sum3/1
  Random Number3/1 -> Sum4/2
  Sum4/1 -> RED_IMU_R1/1
  "x_dot -> x2"/1(dy(t)/dt) -> Sum2/1
  Demux1/8 -> "x_dot -> x1"/1(y(t)), RED_Vy1/1
  Demux1/10 -> Data Store Write6/1
  Demux1/12 -> Data Store Write8/1
  Delay/1 -> Coriolis Function/1(x), "Inertia Function "/1(x), Dynamics Model/1(x)
  "Inertia Function "/1(InertiaS) -> Dynamics Model/2(InertiaS)
  Coriolis Function/1(CoriolisS) -> Dynamics Model/3(CoriolisS)
  Dynamics Model/1(xdot) -> Acceleration to Velocity/1
  Acceleration to Velocity/1 -> Delay/1, Demux1/1
  MATLAB Function/1(Shoulder_Torque) -> Mux1/4
  MATLAB Function/2(Elbow_Torque) -> Mux1/5
  MATLAB Function/3(Wrist_Torque) -> Mux1/6
  Data Store Read5/1 -> MATLAB Function/1(Control_Mode)
  Data Store Read2/1 -> MATLAB Function/2(Shoulder_Command)
  Data Store Read3/1 -> MATLAB Function/3(Elbow_Command)
  Data Store Read4/1 -> MATLAB Function/4(Wrist_Command)
  Data Store Read7/1 -> MATLAB Function/7(Wrist_Angle)
  Data Store Read6/1 -> MATLAB Function/6(Elbow_Angle)
  Data Store Read/1 -> MATLAB Function/5(Shoulder_Angle)
